simulink model "CF010A_GmTqArbn"  (R2013b)
settings: Solver=FixedStepDiscrete  SolverMode=SingleTasking  StartTime=0.0  StopTime=1  FixedStep=0.002  RelTol=1e-3
values from neighbouring files (symbols this model uses):
  ARCHGLBPRM_2MILLISEC_SEC_F32 = DataDict.Constant    [CF010A_GmTqArbn_DataDict.m]
  ESCCMDACTV_CNT_U08 = DataDict.Constant    [CF010A_GmTqArbn_DataDict.m]
  ESCCMDTMPLIMD_CNT_U08 = DataDict.Constant    [CF010A_GmTqArbn_DataDict.m]
  ESCTQCMDOVRLLIM_HWNWTMTR_F32 = DataDict.Constant    [CF010A_GmTqArbn_DataDict.m]
  FINALSLEWLWRLIM_HWNWTMTRPERSEC_F32 = DataDict.Constant    [CF010A_GmTqArbn_DataDict.m]
  GmTqArbnApaAssiScaEna = DataDict.Calibration    [CF010A_GmTqArbn_DataDict.m]
  GmTqArbnApaDampgScaEna = DataDict.Calibration    [CF010A_GmTqArbn_DataDict.m]
  GmTqArbnApaEnaRate = DataDict.Calibration    [CF010A_GmTqArbn_DataDict.m]
  GmTqArbnApaRtnScaEna = DataDict.Calibration    [CF010A_GmTqArbn_DataDict.m]
  GmTqArbnEscMaxTq = DataDict.Calibration    [CF010A_GmTqArbn_DataDict.m]
  GmTqArbnLkaSlewEna = DataDict.Calibration    [CF010A_GmTqArbn_DataDict.m]
  HWTQCMDOVRLLIM_HWNWTMTR_F32 = DataDict.Constant    [CF010A_GmTqArbn_DataDict.m]
  LKACMDHILIM_HWNWTMTR_F32 = DataDict.Constant    [CF010A_GmTqArbn_DataDict.m]
  LKASTACTV_CNT_U08 = DataDict.Constant    [CF010A_GmTqArbn_DataDict.m]
  LKATQCMDOVRLLIM_HWNWTMTR_F32 = DataDict.Constant    [CF010A_GmTqArbn_DataDict.m]
  MOTTQCMDOVRLLIM_MOTNWTMTR_F32 = DataDict.Constant    [CF010A_GmTqArbn_DataDict.m]
  OUTPCMDHILIM_ULS_F32 = DataDict.Constant    [CF010A_GmTqArbn_DataDict.m]
  OUTPCMDLOWRLIM_ULS_F32 = DataDict.Constant    [CF010A_GmTqArbn_DataDict.m]
  POSNSERVOSMOOTHMINLWRLIM_ULSPERSEC_F32 = DataDict.Constant    [CF010A_GmTqArbn_DataDict.m]
  VELDPTTQOVRLMTRCOFFS_HWNWTMTRPERSEC_F32 = DataDict.Constant    [CF010A_GmTqArbn_DataDict.m]
  VELDPTTQOVRLMTRCTQPERVEHSPD_HWNWTMTRPERSECPERKPH_F32 = DataDict.Constant    [CF010A_GmTqArbn_DataDict.m]
libraries: NxtrLim x11, NexteerUtilities x8, FixdToFloat x3, Fil x2, NxtrAbslt x2, simulink x2
(part 1 of 4)
Description:
  | Torque arbitrator module for overlays for GM applications.
  |      This module uses the signals from external modules, other functions, and enable flags from the GMOSH
  |         to determine the amount of input and output torque overlay to apply to SF-01 and SF-04, respectively, and
  |         the amount of scaling to apply to Assist, Return, and Damping.
settings Model: CovMetricSettings=dcmow  CovHTMLOptions=-sRT=1 -aTS=1 -bRG=1 -bTC=1 -hTR=0 -nFC=0 -scm=1 -bcm=1 -xEv=0  covSaveCumulativeToWorkspaceVar=off  CovSaveSingleToWorkspaceVar=off  CovCumulativeReport=on  Creator=HZ32RQ  LastModifiedBy=DZ1YRM
settings SolverCC: AutoInsertRateTranBlk=on  InsertRTBMode=Always
settings DataIOCC: LimitDataPoints=off  SaveFormat=Structure  ReturnWorkspaceOutputs=on
settings OptimizationCC: BlockReduction=off  InlineParams=on  ZeroExternalMemoryAtStartup=off  ZeroInternalMemoryAtStartup=off  OptimizeModelRefInitCode=on  LifeSpan=1
settings DebuggingCC: SignalInfNanChecking=error  SignalRangeChecking=warning  UnderspecifiedInitializationDetection=Simplified  SolverPrmCheckMsg=error  InheritedTsInSrcMsg=error  DiscreteInheritContinuousMsg=error  SingleTaskRateTransMsg=error  TasksWithSamePriorityMsg=error  SigSpecEnsureSampleTimeMsg=error  CheckMatrixSingularityMsg=error  ParameterUnderflowMsg=error  ParameterPrecisionLossMsg=error  ParameterTunabilityLossMsg=error  FixptConstUnderflowMsg=warning  FixptConstOverflowMsg=warning  VectorMatrixConversionMsg=error  SignalLabelMismatchMsg=error  UnconnectedInputMsg=error  UnconnectedOutputMsg=error  UnconnectedLineMsg=error  SFcnCompatibilityMsg=error  UniqueDataStoreMsg=warning  BusObjectLabelMismatch=error  RootOutportRequireBusObject=error  AssertControl=DisableAll  ModelReferenceIOMsg=error  ModelReferenceVersionMismatchMessage=warning  ModelReferenceIOMismatchMessage=error  ModelReferenceCSMismatchMessage=warning  ModelReferenceDataLoggingMessage=error  StateNameClashWarn=warning  StrictBusMsg=ErrorOnBusTreatedAsVector  NonBusSignalsTreatedAsBus=error  SFUnexpectedBacktrackingDiag=error  SFInvalidInputDataAccessInChartInitDiag=error  SFNoUnconditionalDefaultTransitionDiag=error  SFTransitionOutsideNaturalParentDiag=error  SFUnconditionalTransitionShadowingDiag=error  SFUndirectedBroadcastEventsDiag=error
settings ModelReferenceCC: ModelReferenceNumInstancesAllowed=Single
settings RTWCC: SystemTargetFile=autosar.tlc  GenCodeOnly=on  TemplateMakefile=ert_default_tmf  Description=AUTOSAR  GenerateReport=on  ProcessScript=autosar_make_rtw_hook  LaunchReport=on
settings CodeAppCC: GenerateComments=off  IgnoreCustomStorageClasses=off  CustomSymbolStrType=$N$R$M  CustomSymbolStrBlkIO=$N$M  SimulinkBlockComments=off
settings STFCustomTargetCC: ParMdlRefBuildCompliant=on  CompOptLevelCompliant=on  IncludeMdlTerminateFcn=off  CombineOutputUpdateFcns=on  SuppressErrorStatus=on  ERTFirstTimeCompliant=on  ERTCustomFileBanners=on  SupportNonFinite=off  SupportComplex=off  SupportContinuousTime=off  SupportNonInlinedSFcns=off  MATLABClassNameForMDSCustomization=Simulink.SoftwareTarget.ERTCustomization  AutosarCompliant=on  GRTInterface=off  SystemTargetFile=autosar.tlc
settings ERTTargetCC: CodeReplacementLibrary=ANSI_C  ConcurrentExecutionCompliant=off  IncludeMdlTerminateFcn=off  SuppressErrorStatus=on  SupportNonFinite=off  SupportComplex=off  ModelStepFunctionPrototypeControlCompliant=off  CPPClassGenCompliant=off  AutosarCompliant=on  InlinedParameterPlacement=NonHierarchical  ERTCustomFileTemplate=example_file_process.tlc  EnableUserReplacementTypes=on

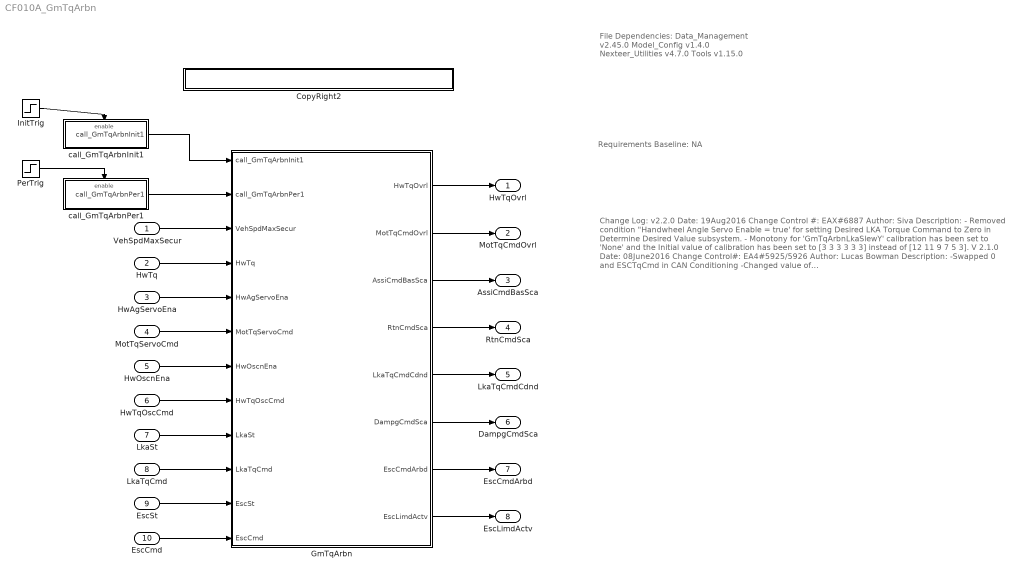
== system CF010A_GmTqArbn ==
  note: File Dependencies:
      |
      | Data_Management v2.45.0
      | Model_Config v1.4.0
      | Nexteer_Utilities v4.7.0
      | Tools v1.15.0
  note: Requirements Baseline: NA
  note: Change Log:
      |
      |
      | v2.2.0
      | Date: 19Aug2016
      | Change Control #: EAX#6887
      | Author: Siva
      | Description:
      | - Removed condition "Handwheel Angle Servo Enable = true' for setting Desired LKA Torque Command to Zero
      |   in Determine Desired Value subsystem.
      | - Monotony for 'GmTqArbnLkaSlewY' calibration has been set to 'None' and the Initial value of calibration has
      |   been set to [3  3  3  3  3  3] instead of [12  11  9  7  5  3].
      |
      |
      | V 2.1.0
      | Date: 08June2016
      | Change Control#: EA4#5925/5926
      | Author: Lucas Bowman
      | Description:
      | -Swapped 0 and ESCTqCmd in CAN Conditioning
      | -Changed value of VELDPTTQOVRLMTRCTQPERVEHSPD_HWNWTMTRPERSECPERKPH_F32 to -7/120
      | -Changed background color in all components to white except for GoTo Flags
      | -Eliminated cross wires and unnecessary GoTo flags
      | -Created labels for wires that are associated with temporary varibles in C file
      |
      | V 2.0.0
      | Date: 04April2016
      | Change Control #: EA4#8765
      | Author: Ting Zhan
      | Description:
      | -Replaced Input signal HwTqOscSt with HwOscnEna
      |
      | V 1.1.0
      | Date: 05Jan2016
      | Change Control #: EA4#3623
      | Author: Hemlata Kamble
      | Description:
      | Following issues mentioned in anomaly CR2143 fixed
      | 1. MtrTqServoSmotngEna name changed to HwAgServoEna
      | and corrected Motor Tq servo command signal name.
      | 2. Trig functions updated for Init and Periodic
      | 3.  PIM Variable name corrected
      | 4. Data type of the Constants used were set to 'double' which
      | are now changed to datatype 'single'
      | 5. Removed incorrect links to requirements in model
      | 6. DD is modified to fix the verify_DD tool errors.
      |
      | V 1.0.0
      | Date: 12Aug2015
      | Change Control #: EA4#1687
      | Author: Qi Wang
      | Description:
      | - Initial release based on EA3 v003
  VehSpdMaxSecur : Inport
  HwTq : Inport  Port=2
  HwAgServoEna : Inport  Port=3
  MotTqServoCmd : Inport  Port=4
  HwOscnEna : Inport  Port=5
  HwTqOscCmd : Inport  RequirementInfo={} %GIDa_71ea23b4_56ba_4dec_a781_aee4be0548fb  Port=6
  LkaSt : Inport  Port=7
  LkaTqCmd : Inport  Port=8
  EscSt : Inport  Port=9
  EscCmd : Inport  Port=10
  CopyRight2 : Subsystem  Description=|  mask(Copyright Information){none=on}
      | Copyright info block.                                               
      |                                                                     
      | Place copyright information at the top of every subsystem in design.
      mask prompts: none "No parameters"
      mask help: Place copyright information at the top of every subsystem in design.
      mask Display:
      | NxtrConf = 'Nexteer Confidential';
      | 
      | sys = bdroot; %handle for the current model ("system")
      | first = get_param(sys,'Created');
      | first = first(end-3:end);  %year is last four digits
      | 
      | last = get_param(sys,'LastModifiedDate');
      | if isempty(last)
      |     last = datestr(now,'yyyy');
      | else
      |     last = last(end-3:end);
      | end
      | 
      | if strcmp(first,last)
      |     fprintf('%s -- Copyright %s Nexteer',NxtrConf,first)
      | else
      |     fprintf('%s -- %s%s- %s Nexteer',NxtrConf,char(169),first,last)
      | end
  GmTqArbn : Subsystem
  InitTrig : Step  Time=0.01  Before=1  After=0  SampleTime=0
  PerTrig : Step  Time=0.01  SampleTime=0
  call_GmTqArbnInit1 : Subsystem  TreatAsAtomicUnit=on
  call_GmTqArbnPer1 : Subsystem  TreatAsAtomicUnit=on
  HwTqOvrl : Outport
  MotTqCmdOvrl : Outport  Port=2
  AssiCmdBasSca : Outport  Port=3
  RtnCmdSca : Outport  Port=4
  LkaTqCmdCdnd : Outport  Port=5
  DampgCmdSca : Outport  Port=6
  EscCmdArbd : Outport  Port=7
  EscLimdActv : Outport  Port=8
  wires:
  VehSpdMaxSecur/1 -> GmTqArbn/3(VehSpdMaxSecur)
  HwTq/1 -> GmTqArbn/4(HwTq)
  HwAgServoEna/1 -> GmTqArbn/5(HwAgServoEna)
  MotTqServoCmd/1 -> GmTqArbn/6(MotTqServoCmd)
  HwOscnEna/1 -> GmTqArbn/7(HwOscnEna)
  HwTqOscCmd/1 -> GmTqArbn/8(HwTqOscCmd)
  LkaSt/1 -> GmTqArbn/9(LkaSt)
  LkaTqCmd/1 -> GmTqArbn/10(LkaTqCmd)
  EscSt/1 -> GmTqArbn/11(EscSt)
  EscCmd/1 -> GmTqArbn/12(EscCmd)
  GmTqArbn/1(HwTqOvrl) -> HwTqOvrl/1
  GmTqArbn/2(MotTqCmdOvrl) -> MotTqCmdOvrl/1
  GmTqArbn/3(AssiCmdBasSca) -> AssiCmdBasSca/1
  GmTqArbn/4(RtnCmdSca) -> RtnCmdSca/1
  GmTqArbn/5(LkaTqCmdCdnd) -> LkaTqCmdCdnd/1
  GmTqArbn/6(DampgCmdSca) -> DampgCmdSca/1
  GmTqArbn/7(EscCmdArbd) -> EscCmdArbd/1
  GmTqArbn/8(EscLimdActv) -> EscLimdActv/1
  call_GmTqArbnInit1/1(call_GmTqArbnInit1) -> GmTqArbn/1(call_GmTqArbnInit1)
  PerTrig/1 -> call_GmTqArbnPer1/Enable
  call_GmTqArbnPer1/1(call_GmTqArbnPer1) -> GmTqArbn/2(call_GmTqArbnPer1)
  InitTrig/1 -> call_GmTqArbnInit1/Enable

== system CF010A_GmTqArbn/CopyRight2 ==

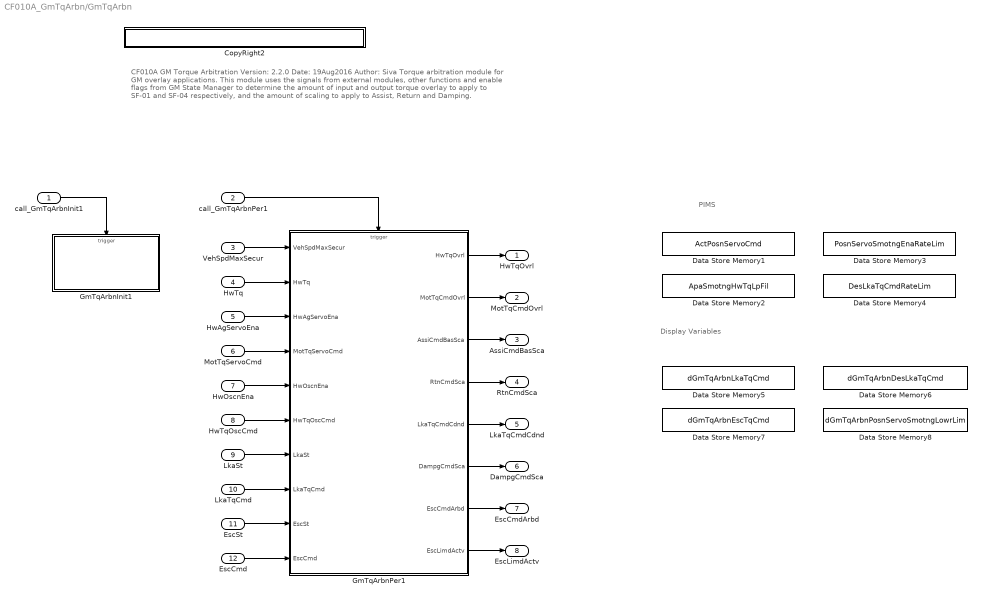
== system CF010A_GmTqArbn/GmTqArbn ==
  note: PIMS
  note: Display Variables
  note: CF010A GM Torque Arbitration
      | Version: 2.2.0      Date: 19Aug2016
      | Author: Siva
      |
      | Torque arbitration module for GM overlay applications.
      | This module uses the signals from external modules, other functions and enable flags from GM State Manager
      | to determine the amount of input and output torque overlay to apply to SF-01 and SF-04 respectively, and the
      | amount of scaling to apply to Assist, Return and Damping.
  call_GmTqArbnInit1 : Inport
  call_GmTqArbnPer1 : Inport  Port=2
  VehSpdMaxSecur : Inport  Port=3
  HwTq : Inport  Port=4
  HwAgServoEna : Inport  Port=5
  MotTqServoCmd : Inport  Port=6
  HwOscnEna : Inport  Port=7
  HwTqOscCmd : Inport  Port=8
  LkaSt : Inport  Port=9
  LkaTqCmd : Inport  Port=10
  EscSt : Inport  Port=11
  EscCmd : Inport  Port=12
  CopyRight2 : Subsystem  Description=|  mask(Copyright Information){none=on}
      | Copyright info block.                                               
      |                                                                     
      | Place copyright information at the top of every subsystem in design.
      mask prompts: none "No parameters"
      mask help: Place copyright information at the top of every subsystem in design.
      mask Display:
      | NxtrConf = 'Nexteer Confidential';
      | 
      | sys = bdroot; %handle for the current model ("system")
      | first = get_param(sys,'Created');
      | first = first(end-3:end);  %year is last four digits
      | 
      | last = get_param(sys,'LastModifiedDate');
      | if isempty(last)
      |     last = datestr(now,'yyyy');
      | else
      |     last = last(end-3:end);
      | end
      | 
      | if strcmp(first,last)
      |     fprintf('%s -- Copyright %s Nexteer',NxtrConf,first)
      | else
      |     fprintf('%s -- %s%s- %s Nexteer',NxtrConf,char(169),first,last)
      | end
  Data Store Memory1 : DataStoreMemory  DataStoreName=ActPosnServoCmd  StateMustResolveToSignalObject=on
  Data Store Memory2 : DataStoreMemory  DataStoreName=ApaSmotngHwTqLpFil  InitialValue=[]  StateMustResolveToSignalObject=on
  Data Store Memory3 : DataStoreMemory  DataStoreName=PosnServoSmotngEnaRateLim  StateMustResolveToSignalObject=on
  Data Store Memory4 : DataStoreMemory  DataStoreName=DesLkaTqCmdRateLim  StateMustResolveToSignalObject=on
  Data Store Memory5 : DataStoreMemory  DataStoreName=dGmTqArbnLkaTqCmd  StateMustResolveToSignalObject=on
  Data Store Memory6 : DataStoreMemory  DataStoreName=dGmTqArbnDesLkaTqCmd  StateMustResolveToSignalObject=on
  Data Store Memory7 : DataStoreMemory  DataStoreName=dGmTqArbnEscTqCmd  StateMustResolveToSignalObject=on
  Data Store Memory8 : DataStoreMemory  DataStoreName=dGmTqArbnPosnServoSmotngLowrLim  StateMustResolveToSignalObject=on
  GmTqArbnInit1 : Subsystem
  GmTqArbnPer1 : Subsystem
  HwTqOvrl : Outport
  MotTqCmdOvrl : Outport  Port=2
  AssiCmdBasSca : Outport  Port=3
  RtnCmdSca : Outport  Port=4
  LkaTqCmdCdnd : Outport  Port=5
  DampgCmdSca : Outport  Port=6
  EscCmdArbd : Outport  Port=7
  EscLimdActv : Outport  Port=8
  wires:
  VehSpdMaxSecur/1 -> GmTqArbnPer1/1(VehSpdMaxSecur)
  HwTq/1 -> GmTqArbnPer1/2(HwTq)
  HwAgServoEna/1 -> GmTqArbnPer1/3(HwAgServoEna)
  MotTqServoCmd/1 -> GmTqArbnPer1/4(MotTqServoCmd)
  HwOscnEna/1 -> GmTqArbnPer1/5(HwOscnEna)
  HwTqOscCmd/1 -> GmTqArbnPer1/6(HwTqOscCmd)
  LkaSt/1 -> GmTqArbnPer1/7(LkaSt)
  LkaTqCmd/1 -> GmTqArbnPer1/8(LkaTqCmd)
  EscSt/1 -> GmTqArbnPer1/9(EscSt)
  EscCmd/1 -> GmTqArbnPer1/10(EscCmd)
  GmTqArbnPer1/1(HwTqOvrl) -> HwTqOvrl/1
  GmTqArbnPer1/2(MotTqCmdOvrl) -> MotTqCmdOvrl/1
  GmTqArbnPer1/3(AssiCmdBasSca) -> AssiCmdBasSca/1
  GmTqArbnPer1/4(RtnCmdSca) -> RtnCmdSca/1
  GmTqArbnPer1/5(LkaTqCmdCdnd) -> LkaTqCmdCdnd/1
  GmTqArbnPer1/6(DampgCmdSca) -> DampgCmdSca/1
  GmTqArbnPer1/7(EscCmdArbd) -> EscCmdArbd/1
  GmTqArbnPer1/8(EscLimdActv) -> EscLimdActv/1
  call_GmTqArbnPer1/1 -> GmTqArbnPer1/Trigger
  call_GmTqArbnInit1/1 -> GmTqArbnInit1/Trigger

== system CF010A_GmTqArbn/call_GmTqArbnInit1 ==
  Enable : EnablePort
  FunctionCallGenerator : simulink/Ports & Subsystems/Function-Call Generator  sample_time=.002  numberOfIterations=1
  Subsystem5 : Subsystem  Description=|  mask(Copyright Information){none=on}
      | Copyright info block.                                               
      |                                                                     
      | Place copyright information at the top of every subsystem in design.
      mask prompts: none "No parameters"
      mask help: Place copyright information at the top of every subsystem in design.
      mask Display:
      | NxtrConf = 'Nexteer Confidential';
      | 
      | sys = bdroot; %handle for the current model ("system")
      | first = get_param(sys,'Created');
      | first = first(end-3:end);  %year is last four digits
      | 
      | last = get_param(sys,'LastModifiedDate');
      | if isempty(last)
      |     last = datestr(now,'yyyy');
      | else
      |     last = last(end-3:end);
      | end
      | 
      | if strcmp(first,last)
      |     fprintf('%s -- Copyright %s Nexteer',NxtrConf,first)
      | else
      |     fprintf('%s -- %s%s- %s Nexteer',NxtrConf,char(169),first,last)
      | end
  call_GmTqArbnInit1 : Outport
  wires:
  FunctionCallGenerator/1 -> call_GmTqArbnInit1/1

== system CF010A_GmTqArbn/call_GmTqArbnPer1 ==
  Enable : EnablePort
  FunctionCallGenerator : simulink/Ports & Subsystems/Function-Call Generator  sample_time=.002  numberOfIterations=1
  Subsystem5 : Subsystem  Description=|  mask(Copyright Information){none=on}
      | Copyright info block.                                               
      |                                                                     
      | Place copyright information at the top of every subsystem in design.
      mask prompts: none "No parameters"
      mask help: Place copyright information at the top of every subsystem in design.
      mask Display:
      | NxtrConf = 'Nexteer Confidential';
      | 
      | sys = bdroot; %handle for the current model ("system")
      | first = get_param(sys,'Created');
      | first = first(end-3:end);  %year is last four digits
      | 
      | last = get_param(sys,'LastModifiedDate');
      | if isempty(last)
      |     last = datestr(now,'yyyy');
      | else
      |     last = last(end-3:end);
      | end
      | 
      | if strcmp(first,last)
      |     fprintf('%s -- Copyright %s Nexteer',NxtrConf,first)
      | else
      |     fprintf('%s -- %s%s- %s Nexteer',NxtrConf,char(169),first,last)
      | end
  call_GmTqArbnPer1 : Outport
  wires:
  FunctionCallGenerator/1 -> call_GmTqArbnPer1/1

== system CF010A_GmTqArbn/GmTqArbn/CopyRight2 ==

== system CF010A_GmTqArbn/GmTqArbn/GmTqArbnInit1 ==
  function : TriggerPort  TriggerType=function-call
  ApaSmotngHwTqLoPassFil : Fil/FilLpInit  Ic=0  Ts=ARCHGLBPRM_2MILLISEC_SEC_F32  Freq=GmTqArbnApaSmotngHwTqLpFilFrq  StVar=ApaSmotngHwTqLpFil
  CopyRight2 : Subsystem  Description=|  mask(Copyright Information){none=on}
      | Copyright info block.                                               
      |                                                                     
      | Place copyright information at the top of every subsystem in design.
      mask prompts: none "No parameters"
      mask help: Place copyright information at the top of every subsystem in design.
      mask Display:
      | NxtrConf = 'Nexteer Confidential';
      | 
      | sys = bdroot; %handle for the current model ("system")
      | first = get_param(sys,'Created');
      | if(isempty(first))
      |     first = datestr(now,'yyyy');
      | else
      |     first = first(end-3:end);  %year is last four digits
      | end
      | 
      | last = get_param(sys,'LastModifiedDate');
      | if isempty(last)
      |     last = datestr(now,'yyyy');
      | else
      |     last = last(end-3:end);
      | end
      | 
      | if strcmp(first,last)
      |     fprintf('%s -- Copyright %s Nexteer',NxtrConf,first)
      | else
      |     fprintf('%s -- %s%s- %s Nexteer',NxtrConf,char(169),first,last)
      | end

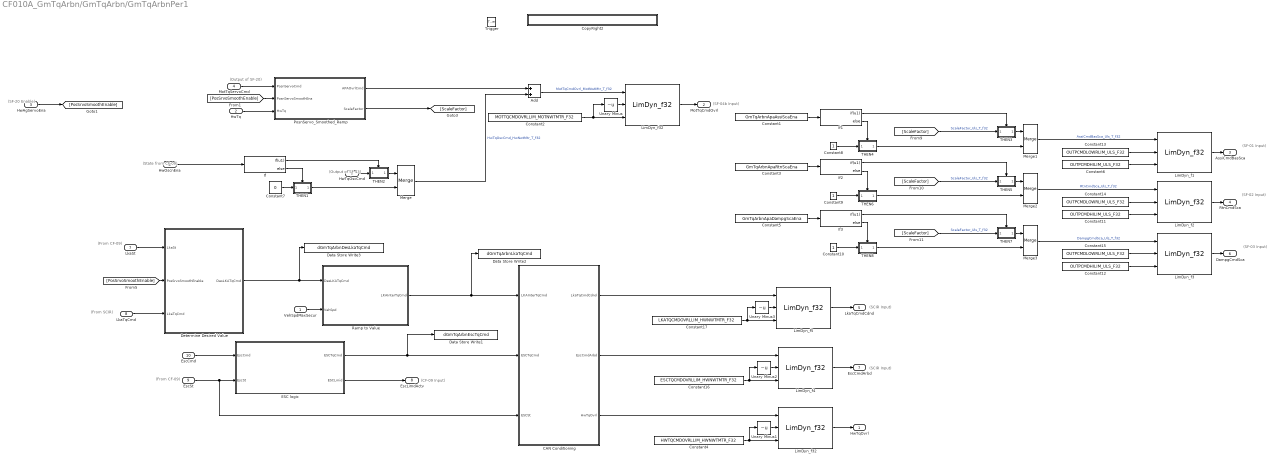
== system CF010A_GmTqArbn/GmTqArbn/GmTqArbnPer1 ==
  note: (SCIR Input)
  note: (SCIR Input)
  note: (SF-03 Input)
  note: (SF-02 Input)
  note: (SF-01 Input)
  note: (SF-04b Input)
  note: (From SCIR)
  note: (From CF-09)
  note: (From CF-09)
  note: (CF-09 Input)
  note: (State from CF-09)
  note: (Output of SF-20)
  note: (SF-20 Enable)
  note: (Output of SF-43)
  VehSpdMaxSecur : Inport
  HwTq : Inport  Port=2
  HwAgServoEna : Inport  Port=3
  MotTqServoCmd : Inport  Port=4
  HwOscnEna : Inport  Port=5
  HwTqOscCmd : Inport  Port=6
  LkaSt : Inport  Port=7
  LkaTqCmd : Inport  Port=8
  EscSt : Inport  Port=9
  EscCmd : Inport  Port=10
  Trigger : TriggerPort  TriggerType=function-call  PortDimensions=1
  Add : Sum
  CAN Conditioning : Subsystem
  Constant1 : Constant  Value=GmTqArbnApaAssiScaEna
  Constant10 : Constant  OutDataTypeStr=single
  Constant11 : Constant  Value=OUTPCMDHILIM_ULS_F32
  Constant12 : Constant  Value=OUTPCMDHILIM_ULS_F32
  Constant13 : Constant  Value=OUTPCMDLOWRLIM_ULS_F32
  Constant14 : Constant  Value=OUTPCMDLOWRLIM_ULS_F32
  Constant15 : Constant  Value=OUTPCMDLOWRLIM_ULS_F32
  Constant16 : Constant  Value=ESCTQCMDOVRLLIM_HWNWTMTR_F32
  Constant17 : Constant  Value=LKATQCMDOVRLLIM_HWNWTMTR_F32
  Constant2 : Constant  Value=MOTTQCMDOVRLLIM_MOTNWTMTR_F32
  Constant3 : Constant  Value=GmTqArbnApaRtnScaEna
  Constant4 : Constant  Value=HWTQCMDOVRLLIM_HWNWTMTR_F32
  Constant5 : Constant  Value=GmTqArbnApaDampgScaEna
  Constant6 : Constant  Value=OUTPCMDHILIM_ULS_F32
  Constant7 : Constant  Value=0  OutDataTypeStr=single
  Constant8 : Constant  OutDataTypeStr=single
  Constant9 : Constant  OutDataTypeStr=single
  CopyRight2 : Subsystem  Description=|  mask(Copyright Information){none=on}
      | Copyright info block.                                               
      |                                                                     
      | Place copyright information at the top of every subsystem in design.
      mask prompts: none "No parameters"
      mask help: Place copyright information at the top of every subsystem in design.
      mask Display:
      | NxtrConf = 'Nexteer Confidential';
      | 
      | sys = bdroot; %handle for the current model ("system")
      | first = get_param(sys,'Created');
      | first = first(end-3:end);  %year is last four digits
      | 
      | last = get_param(sys,'LastModifiedDate');
      | if isempty(last)
      |     last = datestr(now,'yyyy');
      | else
      |     last = last(end-3:end);
      | end
      | 
      | if strcmp(first,last)
      |     fprintf('%s -- Copyright %s Nexteer',NxtrConf,first)
      | else
      |     fprintf('%s -- %s%s- %s Nexteer',NxtrConf,char(169),first,last)
      | end
  Data Store Write1 : DataStoreWrite  DataStoreName=dGmTqArbnEscTqCmd
  Data Store Write2 : DataStoreWrite  DataStoreName=dGmTqArbnLkaTqCmd
  Data Store Write3 : DataStoreWrite  DataStoreName=dGmTqArbnDesLkaTqCmd
  Determine Desired Value : Subsystem
  ESC logic : Subsystem
  If{,1..3} (4 alike) : If  IfExpression=u1
  LimDyn_f{1..5,32} (6 alike) : NxtrLim/LimDyn_f32
  "LimDyn_f32 " : NxtrLim/LimDyn_f32
  Merge{,1..3} (4 alike) : Merge
  PosnServo_Smoothed_Ramp : Subsystem
  Ramp to Value : Subsystem
  THEN1 : Subsystem  RequirementInfo={} %GIDa_b260fa9c_4cdb_4aaa_ae2f_69ac7f8b672c  TreatAsAtomicUnit=on  mask(pass thru, version Nov 30, 2012){nIn=1}
      mask prompts: nIn "Number of input signals"
      mask help:
      | This block passes its input straight through without modification.
      |
      | Enter the number of signals to pass through (integer 1 to 5).
      mask Callback nIn:
      | thisBlock = gcb;
      | a = get_param(thisBlock,'MaskValues');
      | b = cell2mat(a);
      | c = str2num(b);
      | 
      | if c<1 c=1; end
      | if c>5 c=5; end
      | 
      | for idx=1:c
      |     sIdx = num2str(idx);
      |     oldblock = [thisBlock '/In' sIdx];
      |     if strcmp(get_param(oldblock,'BlockType'),'Ground')
      |          newblock = 'built-in/Inport';
      |         pos = get_param(oldblock,'Position');
      |         orient = get_param(oldblock,'Orientation');
      |         delete_block(oldblock);
      |         add_block(newblock,oldblock,'Position',pos, 'Orientation',orient);
      |     end
      | 
      |     oldblock = [thisBlock '/Out' sIdx];
      |     if strcmp(get_param(oldblock,'BlockType'),'Terminator')
      |         newblock = 'built-in/Outport';
      |         pos = get_param(oldblock,'Position');
      |         orient = get_param(oldblock,'Orientation');
      |         delete_block(oldblock);
      |         add_block(newblock,oldblock,'Position',pos, 'Orientation',orient);
      |     end
      | end
      | 
      | for idx=c+1:5
      |     sIdx = num2str(idx);
      |     oldblock = [thisBlock '/In' sIdx];
      |     if strcmp(get_param(oldblock,'BlockType'),'Inport')
      |         newblock = 'built-in/Ground';
      |         pos = get_param(oldblock,'Position');
      |         orient = get_param(oldblock,'Orientation');
      |         delete_block(oldblock);
      |         add_block(newblock,oldblock,'Position',pos, 'Orientation',orient);
      |     end
      | 
      |     oldblock = [thisBlock '/Out' sIdx];
      |     if strcmp(get_param(oldblock,'BlockType'),'Outport')
      |         newblock = 'built-in/Terminator';
      |         pos = get_param(oldblock,'Position');
      |         orient = get_param(oldblock,'Orientation');
      |         delete_block(oldblock);
      |         add_block(newblock,oldblock,'Position',pos, 'Orientation',orient);
      |     end
      | end
      | 
      | 
      | 
      | clear thisBlock oldblock newblock orient pos a b c idx sIdx ;
      mask Display: fprintf('pass\nthru')
  THEN2 : Subsystem  RequirementInfo={} %GIDa_5bde3786_d9f4_4ae5_940c_87d032de86d5  TreatAsAtomicUnit=on  mask(pass thru, version Nov 30, 2012){nIn=1}
      mask prompts: nIn "Number of input signals"
      mask help:
      | This block passes its input straight through without modification.
      |
      | Enter the number of signals to pass through (integer 1 to 5).
      mask Callback nIn:
      | thisBlock = gcb;
      | a = get_param(thisBlock,'MaskValues');
      | b = cell2mat(a);
      | c = str2num(b);
      | 
      | if c<1 c=1; end
      | if c>5 c=5; end
      | 
      | for idx=1:c
      |     sIdx = num2str(idx);
      |     oldblock = [thisBlock '/In' sIdx];
      |     if strcmp(get_param(oldblock,'BlockType'),'Ground')
      |          newblock = 'built-in/Inport';
      |         pos = get_param(oldblock,'Position');
      |         orient = get_param(oldblock,'Orientation');
      |         delete_block(oldblock);
      |         add_block(newblock,oldblock,'Position',pos, 'Orientation',orient);
      |     end
      | 
      |     oldblock = [thisBlock '/Out' sIdx];
      |     if strcmp(get_param(oldblock,'BlockType'),'Terminator')
      |         newblock = 'built-in/Outport';
      |         pos = get_param(oldblock,'Position');
      |         orient = get_param(oldblock,'Orientation');
      |         delete_block(oldblock);
      |         add_block(newblock,oldblock,'Position',pos, 'Orientation',orient);
      |     end
      | end
      | 
      | for idx=c+1:5
      |     sIdx = num2str(idx);
      |     oldblock = [thisBlock '/In' sIdx];
      |     if strcmp(get_param(oldblock,'BlockType'),'Inport')
      |         newblock = 'built-in/Ground';
      |         pos = get_param(oldblock,'Position');
      |         orient = get_param(oldblock,'Orientation');
      |         delete_block(oldblock);
      |         add_block(newblock,oldblock,'Position',pos, 'Orientation',orient);
      |     end
      | 
      |     oldblock = [thisBlock '/Out' sIdx];
      |     if strcmp(get_param(oldblock,'BlockType'),'Outport')
      |         newblock = 'built-in/Terminator';
      |         pos = get_param(oldblock,'Position');
      |         orient = get_param(oldblock,'Orientation');
      |         delete_block(oldblock);
      |         add_block(newblock,oldblock,'Position',pos, 'Orientation',orient);
      |     end
      | end
      | 
      | 
      | 
      | clear thisBlock oldblock newblock orient pos a b c idx sIdx ;
      mask Display: fprintf('pass\nthru')
  THEN3 : Subsystem  RequirementInfo={} %GIDa_d758718b_0144_4eac_9881_31401cf36d2a  TreatAsAtomicUnit=on  mask(pass thru, version Nov 30, 2012){nIn=1}
      mask prompts: nIn "Number of input signals"
      mask help:
      | This block passes its input straight through without modification.
      |
      | Enter the number of signals to pass through (integer 1 to 5).
      mask Callback nIn:
      | thisBlock = gcb;
      | a = get_param(thisBlock,'MaskValues');
      | b = cell2mat(a);
      | c = str2num(b);
      | 
      | if c<1 c=1; end
      | if c>5 c=5; end
      | 
      | for idx=1:c
      |     sIdx = num2str(idx);
      |     oldblock = [thisBlock '/In' sIdx];
      |     if strcmp(get_param(oldblock,'BlockType'),'Ground')
      |          newblock = 'built-in/Inport';
      |         pos = get_param(oldblock,'Position');
      |         orient = get_param(oldblock,'Orientation');
      |         delete_block(oldblock);
      |         add_block(newblock,oldblock,'Position',pos, 'Orientation',orient);
      |     end
      | 
      |     oldblock = [thisBlock '/Out' sIdx];
      |     if strcmp(get_param(oldblock,'BlockType'),'Terminator')
      |         newblock = 'built-in/Outport';
      |         pos = get_param(oldblock,'Position');
      |         orient = get_param(oldblock,'Orientation');
      |         delete_block(oldblock);
      |         add_block(newblock,oldblock,'Position',pos, 'Orientation',orient);
      |     end
      | end
      | 
      | for idx=c+1:5
      |     sIdx = num2str(idx);
      |     oldblock = [thisBlock '/In' sIdx];
      |     if strcmp(get_param(oldblock,'BlockType'),'Inport')
      |         newblock = 'built-in/Ground';
      |         pos = get_param(oldblock,'Position');
      |         orient = get_param(oldblock,'Orientation');
      |         delete_block(oldblock);
      |         add_block(newblock,oldblock,'Position',pos, 'Orientation',orient);
      |     end
      | 
      |     oldblock = [thisBlock '/Out' sIdx];
      |     if strcmp(get_param(oldblock,'BlockType'),'Outport')
      |         newblock = 'built-in/Terminator';
      |         pos = get_param(oldblock,'Position');
      |         orient = get_param(oldblock,'Orientation');
      |         delete_block(oldblock);
      |         add_block(newblock,oldblock,'Position',pos, 'Orientation',orient);
      |     end
      | end
      | 
      | 
      | 
      | clear thisBlock oldblock newblock orient pos a b c idx sIdx ;
      mask Display: fprintf('pass\nthru')
  THEN4 : Subsystem  RequirementInfo={} %GIDa_e1ba3c2d_8fad_48f0_b475_5acb6897d40c  TreatAsAtomicUnit=on  mask(pass thru, version Nov 30, 2012){nIn=1}
      mask prompts: nIn "Number of input signals"
      mask help:
      | This block passes its input straight through without modification.
      |
      | Enter the number of signals to pass through (integer 1 to 5).
      mask Callback nIn:
      | thisBlock = gcb;
      | a = get_param(thisBlock,'MaskValues');
      | b = cell2mat(a);
      | c = str2num(b);
      | 
      | if c<1 c=1; end
      | if c>5 c=5; end
      | 
      | for idx=1:c
      |     sIdx = num2str(idx);
      |     oldblock = [thisBlock '/In' sIdx];
      |     if strcmp(get_param(oldblock,'BlockType'),'Ground')
      |          newblock = 'built-in/Inport';
      |         pos = get_param(oldblock,'Position');
      |         orient = get_param(oldblock,'Orientation');
      |         delete_block(oldblock);
      |         add_block(newblock,oldblock,'Position',pos, 'Orientation',orient);
      |     end
      | 
      |     oldblock = [thisBlock '/Out' sIdx];
      |     if strcmp(get_param(oldblock,'BlockType'),'Terminator')
      |         newblock = 'built-in/Outport';
      |         pos = get_param(oldblock,'Position');
      |         orient = get_param(oldblock,'Orientation');
      |         delete_block(oldblock);
      |         add_block(newblock,oldblock,'Position',pos, 'Orientation',orient);
      |     end
      | end
      | 
      | for idx=c+1:5
      |     sIdx = num2str(idx);
      |     oldblock = [thisBlock '/In' sIdx];
      |     if strcmp(get_param(oldblock,'BlockType'),'Inport')
      |         newblock = 'built-in/Ground';
      |         pos = get_param(oldblock,'Position');
      |         orient = get_param(oldblock,'Orientation');
      |         delete_block(oldblock);
      |         add_block(newblock,oldblock,'Position',pos, 'Orientation',orient);
      |     end
      | 
      |     oldblock = [thisBlock '/Out' sIdx];
      |     if strcmp(get_param(oldblock,'BlockType'),'Outport')
      |         newblock = 'built-in/Terminator';
      |         pos = get_param(oldblock,'Position');
      |         orient = get_param(oldblock,'Orientation');
      |         delete_block(oldblock);
      |         add_block(newblock,oldblock,'Position',pos, 'Orientation',orient);
      |     end
      | end
      | 
      | 
      | 
      | clear thisBlock oldblock newblock orient pos a b c idx sIdx ;
      mask Display: fprintf('pass\nthru')
  THEN5 : Subsystem  RequirementInfo={} %GIDa_fea473c1_093f_4ff2_899d_9142ecda2b9c  TreatAsAtomicUnit=on  mask(pass thru, version Nov 30, 2012){nIn=1}
      mask prompts: nIn "Number of input signals"
      mask help:
      | This block passes its input straight through without modification.
      |
      | Enter the number of signals to pass through (integer 1 to 5).
      mask Callback nIn:
      | thisBlock = gcb;
      | a = get_param(thisBlock,'MaskValues');
      | b = cell2mat(a);
      | c = str2num(b);
      | 
      | if c<1 c=1; end
      | if c>5 c=5; end
      | 
      | for idx=1:c
      |     sIdx = num2str(idx);
      |     oldblock = [thisBlock '/In' sIdx];
      |     if strcmp(get_param(oldblock,'BlockType'),'Ground')
      |          newblock = 'built-in/Inport';
      |         pos = get_param(oldblock,'Position');
      |         orient = get_param(oldblock,'Orientation');
      |         delete_block(oldblock);
      |         add_block(newblock,oldblock,'Position',pos, 'Orientation',orient);
      |     end
      | 
      |     oldblock = [thisBlock '/Out' sIdx];
      |     if strcmp(get_param(oldblock,'BlockType'),'Terminator')
      |         newblock = 'built-in/Outport';
      |         pos = get_param(oldblock,'Position');
      |         orient = get_param(oldblock,'Orientation');
      |         delete_block(oldblock);
      |         add_block(newblock,oldblock,'Position',pos, 'Orientation',orient);
      |     end
      | end
      | 
      | for idx=c+1:5
      |     sIdx = num2str(idx);
      |     oldblock = [thisBlock '/In' sIdx];
      |     if strcmp(get_param(oldblock,'BlockType'),'Inport')
      |         newblock = 'built-in/Ground';
      |         pos = get_param(oldblock,'Position');
      |         orient = get_param(oldblock,'Orientation');
      |         delete_block(oldblock);
      |         add_block(newblock,oldblock,'Position',pos, 'Orientation',orient);
      |     end
      | 
      |     oldblock = [thisBlock '/Out' sIdx];
      |     if strcmp(get_param(oldblock,'BlockType'),'Outport')
      |         newblock = 'built-in/Terminator';
      |         pos = get_param(oldblock,'Position');
      |         orient = get_param(oldblock,'Orientation');
      |         delete_block(oldblock);
      |         add_block(newblock,oldblock,'Position',pos, 'Orientation',orient);
      |     end
      | end
      | 
      | 
      | 
      | clear thisBlock oldblock newblock orient pos a b c idx sIdx ;
      mask Display: fprintf('pass\nthru')
  THEN6 : Subsystem  RequirementInfo={} %GIDa_0d0ff04e_04bf_43f9_88c4_85e73db6cdf4  TreatAsAtomicUnit=on  mask(pass thru, version Nov 30, 2012){nIn=1}
      mask prompts: nIn "Number of input signals"
      mask help:
      | This block passes its input straight through without modification.
      |
      | Enter the number of signals to pass through (integer 1 to 5).
      mask Callback nIn:
      | thisBlock = gcb;
      | a = get_param(thisBlock,'MaskValues');
      | b = cell2mat(a);
      | c = str2num(b);
      | 
      | if c<1 c=1; end
      | if c>5 c=5; end
      | 
      | for idx=1:c
      |     sIdx = num2str(idx);
      |     oldblock = [thisBlock '/In' sIdx];
      |     if strcmp(get_param(oldblock,'BlockType'),'Ground')
      |          newblock = 'built-in/Inport';
      |         pos = get_param(oldblock,'Position');
      |         orient = get_param(oldblock,'Orientation');
      |         delete_block(oldblock);
      |         add_block(newblock,oldblock,'Position',pos, 'Orientation',orient);
      |     end
      | 
      |     oldblock = [thisBlock '/Out' sIdx];
      |     if strcmp(get_param(oldblock,'BlockType'),'Terminator')
      |         newblock = 'built-in/Outport';
      |         pos = get_param(oldblock,'Position');
      |         orient = get_param(oldblock,'Orientation');
      |         delete_block(oldblock);
      |         add_block(newblock,oldblock,'Position',pos, 'Orientation',orient);
      |     end
      | end
      | 
      | for idx=c+1:5
      |     sIdx = num2str(idx);
      |     oldblock = [thisBlock '/In' sIdx];
      |     if strcmp(get_param(oldblock,'BlockType'),'Inport')
      |         newblock = 'built-in/Ground';
      |         pos = get_param(oldblock,'Position');
      |         orient = get_param(oldblock,'Orientation');
      |         delete_block(oldblock);
      |         add_block(newblock,oldblock,'Position',pos, 'Orientation',orient);
      |     end
      | 
      |     oldblock = [thisBlock '/Out' sIdx];
      |     if strcmp(get_param(oldblock,'BlockType'),'Outport')
      |         newblock = 'built-in/Terminator';
      |         pos = get_param(oldblock,'Position');
      |         orient = get_param(oldblock,'Orientation');
      |         delete_block(oldblock);
      |         add_block(newblock,oldblock,'Position',pos, 'Orientation',orient);
      |     end
      | end
      | 
      | 
      | 
      | clear thisBlock oldblock newblock orient pos a b c idx sIdx ;
      mask Display: fprintf('pass\nthru')
  THEN7 : Subsystem  RequirementInfo={} %GIDa_e8415cb2_c251_4c08_9b19_892187c308a4  TreatAsAtomicUnit=on  mask(pass thru, version Nov 30, 2012){nIn=1}
      mask prompts: nIn "Number of input signals"
      mask help:
      | This block passes its input straight through without modification.
      |
      | Enter the number of signals to pass through (integer 1 to 5).
      mask Callback nIn:
      | thisBlock = gcb;
      | a = get_param(thisBlock,'MaskValues');
      | b = cell2mat(a);
      | c = str2num(b);
      | 
      | if c<1 c=1; end
      | if c>5 c=5; end
      | 
      | for idx=1:c
      |     sIdx = num2str(idx);
      |     oldblock = [thisBlock '/In' sIdx];
      |     if strcmp(get_param(oldblock,'BlockType'),'Ground')
      |          newblock = 'built-in/Inport';
      |         pos = get_param(oldblock,'Position');
      |         orient = get_param(oldblock,'Orientation');
      |         delete_block(oldblock);
      |         add_block(newblock,oldblock,'Position',pos, 'Orientation',orient);
      |     end
      | 
      |     oldblock = [thisBlock '/Out' sIdx];
      |     if strcmp(get_param(oldblock,'BlockType'),'Terminator')
      |         newblock = 'built-in/Outport';
      |         pos = get_param(oldblock,'Position');
      |         orient = get_param(oldblock,'Orientation');
      |         delete_block(oldblock);
      |         add_block(newblock,oldblock,'Position',pos, 'Orientation',orient);
      |     end
      | end
      | 
      | for idx=c+1:5
      |     sIdx = num2str(idx);
      |     oldblock = [thisBlock '/In' sIdx];
      |     if strcmp(get_param(oldblock,'BlockType'),'Inport')
      |         newblock = 'built-in/Ground';
      |         pos = get_param(oldblock,'Position');
      |         orient = get_param(oldblock,'Orientation');
      |         delete_block(oldblock);
      |         add_block(newblock,oldblock,'Position',pos, 'Orientation',orient);
      |     end
      | 
      |     oldblock = [thisBlock '/Out' sIdx];
      |     if strcmp(get_param(oldblock,'BlockType'),'Outport')
      |         newblock = 'built-in/Terminator';
      |         pos = get_param(oldblock,'Position');
      |         orient = get_param(oldblock,'Orientation');
      |         delete_block(oldblock);
      |         add_block(newblock,oldblock,'Position',pos, 'Orientation',orient);
      |     end
      | end
      | 
      | 
      | 
      | clear thisBlock oldblock newblock orient pos a b c idx sIdx ;
      mask Display: fprintf('pass\nthru')
  THEN8 : Subsystem  RequirementInfo={} %GIDa_1c38b251_2d22_4757_b5bd_5c35a9eeaa83  TreatAsAtomicUnit=on  mask(pass thru, version Nov 30, 2012){nIn=1}
      mask prompts: nIn "Number of input signals"
      mask help:
      | This block passes its input straight through without modification.
      |
      | Enter the number of signals to pass through (integer 1 to 5).
      mask Callback nIn:
      | thisBlock = gcb;
      | a = get_param(thisBlock,'MaskValues');
      | b = cell2mat(a);
      | c = str2num(b);
      | 
      | if c<1 c=1; end
      | if c>5 c=5; end
      | 
      | for idx=1:c
      |     sIdx = num2str(idx);
      |     oldblock = [thisBlock '/In' sIdx];
      |     if strcmp(get_param(oldblock,'BlockType'),'Ground')
      |          newblock = 'built-in/Inport';
      |         pos = get_param(oldblock,'Position');
      |         orient = get_param(oldblock,'Orientation');
      |         delete_block(oldblock);
      |         add_block(newblock,oldblock,'Position',pos, 'Orientation',orient);
      |     end
      | 
      |     oldblock = [thisBlock '/Out' sIdx];
      |     if strcmp(get_param(oldblock,'BlockType'),'Terminator')
      |         newblock = 'built-in/Outport';
      |         pos = get_param(oldblock,'Position');
      |         orient = get_param(oldblock,'Orientation');
      |         delete_block(oldblock);
      |         add_block(newblock,oldblock,'Position',pos, 'Orientation',orient);
      |     end
      | end
      | 
      | for idx=c+1:5
      |     sIdx = num2str(idx);
      |     oldblock = [thisBlock '/In' sIdx];
      |     if strcmp(get_param(oldblock,'BlockType'),'Inport')
      |         newblock = 'built-in/Ground';
      |         pos = get_param(oldblock,'Position');
      |         orient = get_param(oldblock,'Orientation');
      |         delete_block(oldblock);
      |         add_block(newblock,oldblock,'Position',pos, 'Orientation',orient);
      |     end
      | 
      |     oldblock = [thisBlock '/Out' sIdx];
      |     if strcmp(get_param(oldblock,'BlockType'),'Outport')
      |         newblock = 'built-in/Terminator';
      |         pos = get_param(oldblock,'Position');
      |         orient = get_param(oldblock,'Orientation');
      |         delete_block(oldblock);
      |         add_block(newblock,oldblock,'Position',pos, 'Orientation',orient);
      |     end
      | end
      | 
      | 
      | 
      | clear thisBlock oldblock newblock orient pos a b c idx sIdx ;
      mask Display: fprintf('pass\nthru')
  Unary Minus{,1..3} (4 alike) : UnaryMinus
  HwTqOvrl : Outport
  MotTqCmdOvrl : Outport  Port=2
  AssiCmdBasSca : Outport  Port=3
  RtnCmdSca : Outport  Port=4
  LkaTqCmdCdnd : Outport  Port=5
  DampgCmdSca : Outport  Port=6
  EscCmdArbd : Outport  Port=7
  EscLimdActv : Outport  Port=8
  wires:
  ESC logic/1(ESCTqCmd) -> Data Store Write1/1, CAN Conditioning/2(ESCTqCmd)
  Constant7/1 -> THEN1/1(In1)
  MotTqServoCmd/1 -> PosnServo_Smoothed_Ramp/1(PosnServoCmd)
  Merge2/1 -> LimDyn_f2/1  "RtnCmdSca_Uls_T_f32"
  EscCmd/1 -> ESC logic/1(EscCmd)
  Merge/1 -> Add/2  "HwTqOscCmd_HwNwtMtr_T_f32"
  Add/1 -> "LimDyn_f32 "/1  "MotTqCmdOvrl_MotNwtMtr_T_f32"
  HwOscnEna/1 -> If/1
  [PosSrvoSmoothEnable] -> PosnServo_Smoothed_Ramp/2(PosnServoSmoothEna)
  CAN Conditioning/1(LkaTqCmdCdnd) -> LimDyn_f5/1
  Determine Desired Value/1(DesLKATqCmd) -> Data Store Write3/1, Ramp to Value/1(DesLKATqCmd)
  [PosSrvoSmoothEnable] -> Determine Desired Value/2(PosSrvoSmoothEnable)
  PosnServo_Smoothed_Ramp/2(ScaleFactor) -> [ScaleFactor]
  Ramp to Value/1(LKAInterTqCmd) -> Data Store Write2/1, CAN Conditioning/1(LKAInterTqCmd)
  LkaSt/1 -> Determine Desired Value/1(LkaSt)
  Constant3/1 -> If2/1
  Constant1/1 -> If1/1
  Merge3/1 -> LimDyn_f3/1  "DampgCmdSca_Uls_T_f32"
  HwTqOscCmd/1 -> THEN2/1(In1)
  LkaTqCmd/1 -> Determine Desired Value/3(LkaTqCmd)
  CAN Conditioning/3(HwTqOvrl) -> LimDyn_f32/1
  ESC logic/2(ESCLmid) -> EscLimdActv/1
  THEN3/1(Out1) -> Merge1/1
  HwTq/1 -> PosnServo_Smoothed_Ramp/3(HwTq)
  HwAgServoEna/1 -> [PosSrvoSmoothEnable]
  Constant5/1 -> If3/1
  PosnServo_Smoothed_Ramp/1(APAOvrlCmd) -> Add/1
  EscSt/1 -> CAN Conditioning/3(ESCSt), ESC logic/2(EscSt)
  CAN Conditioning/2(EscCmdArbd) -> LimDyn_f4/1
  If/2 -> THEN1/Action
  If/1 -> THEN2/Action
  THEN2/1(Out1) -> Merge/1
  THEN1/1(Out1) -> Merge/2
  [ScaleFactor] -> THEN3/1(In1)  "ScaleFactor_Uls_T_f32"
  If1/1 -> THEN3/Action
  Constant8/1 -> THEN4/1(In1)
  If1/2 -> THEN4/Action
  Merge1/1 -> LimDyn_f1/1  "AssiCmdBasSca_Uls_T_f32"
  THEN4/1(Out1) -> Merge1/2
  THEN5/1(Out1) -> Merge2/1
  [ScaleFactor] -> THEN5/1(In1)  "ScaleFactor_Uls_T_f32"
  If2/1 -> THEN5/Action
  Constant9/1 -> THEN6/1(In1)
  If2/2 -> THEN6/Action
  THEN6/1(Out1) -> Merge2/2
  THEN7/1(Out1) -> Merge3/1
  [ScaleFactor] -> THEN7/1(In1)  "ScaleFactor_Uls_T_f32"
  If3/1 -> THEN7/Action
  Constant10/1 -> THEN8/1(In1)
  If3/2 -> THEN8/Action
  THEN8/1(Out1) -> Merge3/2
  "LimDyn_f32 "/1 -> MotTqCmdOvrl/1
  Unary Minus/1 -> "LimDyn_f32 "/2
  Constant2/1 -> "LimDyn_f32 "/3, Unary Minus/1
  Constant4/1 -> LimDyn_f32/3, Unary Minus1/1
  Unary Minus1/1 -> LimDyn_f32/2
  LimDyn_f1/1 -> AssiCmdBasSca/1
  LimDyn_f2/1 -> RtnCmdSca/1
  LimDyn_f3/1 -> DampgCmdSca/1
  Constant6/1 -> LimDyn_f1/3
  Constant11/1 -> LimDyn_f2/3
  Constant12/1 -> LimDyn_f3/3
  Constant13/1 -> LimDyn_f1/2
  Constant14/1 -> LimDyn_f2/2
  Constant15/1 -> LimDyn_f3/2
  LimDyn_f32/1 -> HwTqOvrl/1
  Constant16/1 -> Unary Minus2/1, LimDyn_f4/3
  Unary Minus2/1 -> LimDyn_f4/2
  LimDyn_f4/1 -> EscCmdArbd/1
  Constant17/1 -> LimDyn_f5/3, Unary Minus3/1
  Unary Minus3/1 -> LimDyn_f5/2
  LimDyn_f5/1 -> LkaTqCmdCdnd/1
  VehSpdMaxSecur/1 -> Ramp to Value/2(VehSpd)

== system CF010A_GmTqArbn/call_GmTqArbnInit1/Subsystem5 ==

== system CF010A_GmTqArbn/call_GmTqArbnPer1/Subsystem5 ==

== system CF010A_GmTqArbn/GmTqArbn/GmTqArbnInit1/CopyRight2 ==
